simulink model "gm_HDL_pfc_gold_fi"  (R2024b)
settings: Solver=FixedStepDiscrete  StartTime=0.0  StopTime=.4  RelTol=1e-3
InitFcn:
  | fidelity_pfc_vals;
  | load('C:\Users\Angel\Desktop\hil\pfc3ph\matlab\sim\sschdl\pfc_desktop\stateSpaceParameters.mat');
undefined symbols (not defined in the file or in its folder): a, b, c, Down, tsw, Up
libraries: hdlmdlgenlib x24, simulink x23, hdlsllib x7, eePwmGenerator x3, dspsrcs4 x3, simulink_need_slupdate x1
(part 1 of 3)
settings Model: Creator=angro  LastModifiedBy=Angel
settings OptimizationCC: BlockReduction=off  ConditionallyExecuteInputs=off  DefaultParameterBehavior=Inlined  InheritOutputTypeSmallerThanSingle=on  DefaultUnderspecifiedDataType=single
settings DebuggingCC: SignalRangeChecking=warning  AlgebraicLoopMsg=error  ArtificialAlgebraicLoopMsg=error  InheritedTsInSrcMsg=none  SingleTaskRateTransMsg=error  UnconnectedInputMsg=warning  UnconnectedOutputMsg=warning  UnconnectedLineMsg=warning
settings HardwareCC: ProdBitPerPointer=32  ProdBitPerSizeT=32  ProdBitPerPtrDiffT=32  ProdLargestAtomicFloat=None  ProdIntDivRoundTo=Undefined  ProdEndianess=Unspecified  ProdWordSize=32  ProdHWDeviceType=ASIC/FPGA->ASIC/FPGA  TargetBitPerPointer=64  TargetBitPerSizeT=64  TargetBitPerPtrDiffT=64  TargetLongLongMode=on  TargetIntDivRoundTo=Zero  TargetEndianess=LittleEndian  TargetWordSize=64  TargetHWDeviceType=Custom Processor->MATLAB Host Computer  ProdEqTarget=off

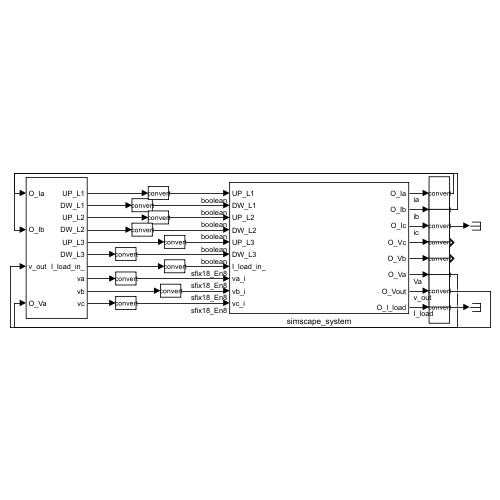
[thumbnail: Simulink's stored preview of the top-level diagram]
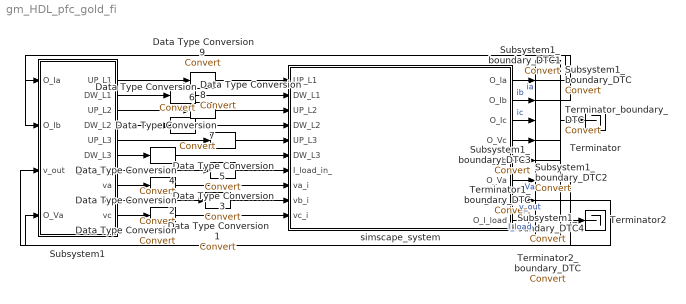
== system gm_HDL_pfc_gold_fi ==
  Data Type Conversion{,1..9} (10 alike) : DataTypeConversion  SaturateOnIntegerOverflow=off  RndMeth=Floor
  Subsystem1 : Subsystem
  Subsystem1_boundary_DTC{,1..4} (5 alike) : DataTypeConversion
  Terminator : Terminator
  Terminator1_boundary_DTC : DataTypeConversion
  Terminator2 : Terminator
  Terminator2_boundary_DTC : DataTypeConversion
  Terminator_boundary_DTC : DataTypeConversion
  simscape_system : Subsystem
  wires:
  Subsystem1_boundary_DTC4/1 -> Subsystem1/4(O_Va)
  Subsystem1_boundary_DTC1/1 -> Subsystem1/2(O_Ib)
  Subsystem1_boundary_DTC/1 -> Subsystem1/1(O_Ia)
  Terminator2_boundary_DTC/1 -> Terminator2/1
  simscape_system/8(O_I_load) -> Terminator2_boundary_DTC/1  "I_load"
  Terminator1_boundary_DTC/1 -> Subsystem1/3(v_out)
  simscape_system/7(O_Vout) -> Terminator1_boundary_DTC/1  "v_out"
  simscape_system/6(O_Va) -> Subsystem1_boundary_DTC4/1  "Va"
  simscape_system/5(O_Vb) -> Subsystem1_boundary_DTC3/1
  simscape_system/4(O_Vc) -> Subsystem1_boundary_DTC2/1
  Terminator_boundary_DTC/1 -> Terminator/1
  simscape_system/3(O_Ic) -> Terminator_boundary_DTC/1  "ic"
  simscape_system/2(O_Ib) -> Subsystem1_boundary_DTC1/1  "ib"
  simscape_system/1(O_Ia) -> Subsystem1_boundary_DTC/1  "ia"
  Data Type Conversion9/1 -> simscape_system/1(UP_L1)
  Data Type Conversion8/1 -> simscape_system/2(DW_L1)
  Data Type Conversion7/1 -> simscape_system/3(UP_L2)
  Data Type Conversion6/1 -> simscape_system/4(DW_L2)
  Data Type Conversion5/1 -> simscape_system/5(UP_L3)
  Data Type Conversion4/1 -> simscape_system/6(DW_L3)
  Data Type Conversion3/1 -> simscape_system/7(I_load_in_)
  Data Type Conversion2/1 -> simscape_system/8(va_i)
  Data Type Conversion1/1 -> simscape_system/9(vb_i)
  Data Type Conversion/1 -> simscape_system/10(vc_i)
  Subsystem1/10(vc) -> Data Type Conversion/1
  Subsystem1/9(vb) -> Data Type Conversion1/1
  Subsystem1/8(va) -> Data Type Conversion2/1
  Subsystem1/6(DW_L3) -> Data Type Conversion4/1
  Subsystem1/5(UP_L3) -> Data Type Conversion5/1
  Subsystem1/4(DW_L2) -> Data Type Conversion6/1
  Subsystem1/3(UP_L2) -> Data Type Conversion7/1
  Subsystem1/2(DW_L1) -> Data Type Conversion8/1
  Subsystem1/1(UP_L1) -> Data Type Conversion9/1
  Subsystem1/7(I_load_in_) -> Data Type Conversion3/1

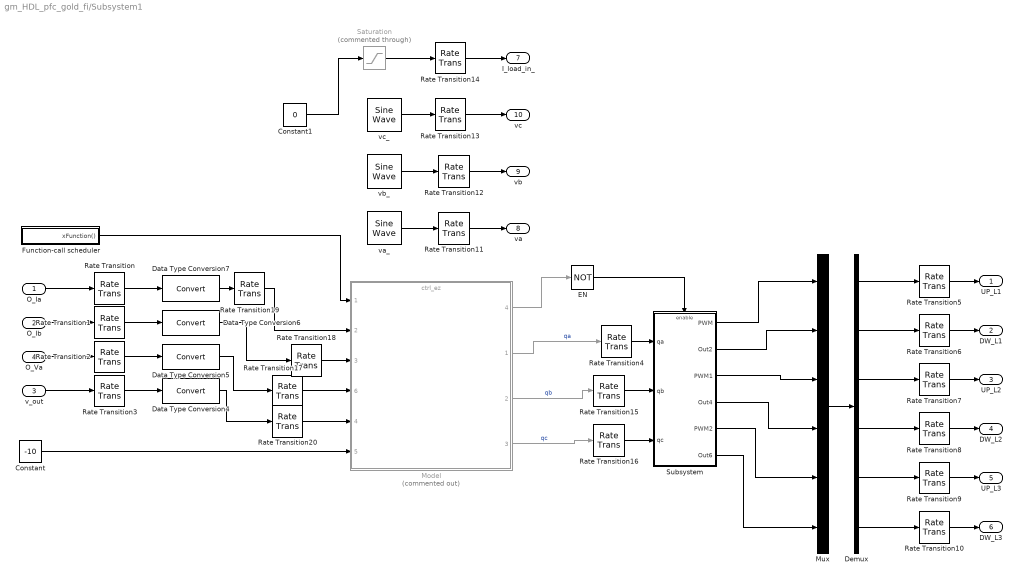
== system gm_HDL_pfc_gold_fi/Subsystem1 ==
  O_Ia : Inport
  O_Ib : Inport  Port=2
  v_out : Inport  Port=3
  O_Va : Inport  Port=4
  Constant : Constant  Value=-10  OutDataTypeStr=single  SampleTime=-1
  Constant1 : Constant  Value=0
  Data Type Conversion{4..7} (4 alike) : DataTypeConversion  SaturateOnIntegerOverflow=off  RndMeth=Floor
  Demux : Demux  Outputs=6
  EN : Logic  Operator=NOT  IconShape=distinctive  AllPortsSameDT=off  OutDataTypeStr=boolean
  Function-call scheduler : Test Sequence  TreatAsAtomicUnit=on  SystemSampleTime=tsw
  Model : ModelReference  Commented=on  ModelNameDialog=ctrl_ez.slx  SimulationMode=Normal  ScheduleRates=on  ModelReferenceVersion=1.93
      settings: PortSchema="{\"entries\":[{\"content\":{\"sides\":[{\"content\":{\"connectorIds\":[\"In1\",\"In2\",\"In3\",\"In6\",\"In4\",\"In5\"]},\"type\":\"ConnectorPlacement.EquallySpacedRectSide\",\"uuid\":\"06228333-cac0-4194-8a9e-b8aeb0f2d2c3\"},{\"content\":{\"connectorIds\":[\"Out4\",\"Out1\",\"Out2\",\"Out3\"],\"side\":\"RIGHT\"},\"type\":\"ConnectorPlacement.EquallySpacedRectSide\",\"uuid\":\"40fc62da-d5d1-4d07-aeb6-22788cb15ec8\"},{\"content\":{\"side\":\"TOP\"},\"type\":\"ConnectorPlacement.EquallySpacedRectSide\",\"uuid\":\"88200490-c98c-4a0a-a21b-c8f9cef9ee2d\"}]},\"type\":\"ConnectorPlacement.EquallySpacedConnector\",\"uuid\":\"5f40978a-c38c-41d1-a6a1-03264eebf395\"}],\"packageUris\":[\"http://schema.mathworks.com/mf0/Connector/R2020b\"],\"version\":\"1.0\"}"
  Mux : Mux  Inputs=6
  Rate Transition{,1..3,14} (5 alike) : RateTransition  OutPortSampleTime=t_ss
  Rate Transition{4..13,15..20} (16 alike) : RateTransition
  Saturation : Saturate  Commented=through  UpperLimit=3
  Subsystem : Subsystem
  va_ : dspsrcs4/Sine Wave  Amplitude=325  Frequency=50  Phase=0  SampleMode=Discrete  OutComplex=Real  CompMethod=Table lookup  TableSize=Speed  SampleTime=tsw  SamplesPerFrame=1  ResetState=Restart at time zero  OutputFrames=off  dataType=double  wordLen=16  udDataType=sfix(16)  fracBitsMode=Best precision  numFracBits=15  OutDataTypeStr=double  LastOutDataTypeStr=double
  vb_ : dspsrcs4/Sine Wave  Amplitude=325  Frequency=50  Phase=(-2*pi/3)  SampleMode=Discrete  OutComplex=Real  CompMethod=Table lookup  TableSize=Speed  SampleTime=tsw  SamplesPerFrame=1  ResetState=Restart at time zero  OutputFrames=off  dataType=double  wordLen=16  udDataType=sfix(16)  fracBitsMode=Best precision  numFracBits=15  OutDataTypeStr=double  LastOutDataTypeStr=double
  vc_ : dspsrcs4/Sine Wave  Amplitude=325  Frequency=50  Phase=(2*pi/3)  SampleMode=Discrete  OutComplex=Real  CompMethod=Table lookup  TableSize=Speed  SampleTime=tsw  SamplesPerFrame=1  ResetState=Restart at time zero  OutputFrames=off  dataType=double  wordLen=16  udDataType=sfix(16)  fracBitsMode=Best precision  numFracBits=15  OutDataTypeStr=double  LastOutDataTypeStr=double
  UP_L1 : Outport
  DW_L1 : Outport  Port=2
  UP_L2 : Outport  Port=3
  DW_L2 : Outport  Port=4
  UP_L3 : Outport  Port=5
  DW_L3 : Outport  Port=6
  I_load_in_ : Outport  Port=7
  va : Outport  Port=8
  vb : Outport  Port=9
  vc : Outport  Port=10
  wires:
  Rate Transition20/1 -> Model/4
  Rate Transition17/1 -> Model/6
  Rate Transition18/1 -> Model/3
  Rate Transition19/1 -> Model/2
  Rate Transition16/1 -> Subsystem/3(qc)
  Rate Transition15/1 -> Subsystem/2(qb)
  Rate Transition4/1 -> Subsystem/1(qa)
  EN/1 -> Subsystem/Enable
  Model/4 -> EN/1
  Subsystem/6(Out6) -> Mux/6
  Subsystem/5(PWM2) -> Mux/5
  Subsystem/4(Out4) -> Mux/4
  Subsystem/3(PWM1) -> Mux/3
  Subsystem/2(Out2) -> Mux/2
  Subsystem/1(PWM) -> Mux/1
  Model/3 -> Rate Transition16/1  "qc"
  Model/2 -> Rate Transition15/1  "qb"
  Model/1 -> Rate Transition4/1  "qa"
  Mux/1 -> Demux/1
  Function-call scheduler/1(xFunction()) -> Model/1
  Constant1/1 -> Saturation/1
  Constant/1 -> Model/5
  Data Type Conversion4/1 -> Rate Transition20/1
  Data Type Conversion5/1 -> Rate Transition17/1
  Data Type Conversion6/1 -> Rate Transition18/1
  Data Type Conversion7/1 -> Rate Transition19/1
  Rate Transition2/1 -> Data Type Conversion5/1
  Rate Transition1/1 -> Data Type Conversion6/1
  Rate Transition/1 -> Data Type Conversion7/1
  Rate Transition3/1 -> Data Type Conversion4/1
  Rate Transition7/1 -> UP_L2/1
  Demux/6 -> Rate Transition10/1
  Demux/2 -> Rate Transition6/1
  Demux/1 -> Rate Transition5/1
  Rate Transition5/1 -> UP_L1/1
  Rate Transition9/1 -> UP_L3/1
  Rate Transition13/1 -> vc/1
  Rate Transition8/1 -> DW_L2/1
  Demux/3 -> Rate Transition7/1
  Demux/4 -> Rate Transition8/1
  Rate Transition11/1 -> va/1
  Demux/5 -> Rate Transition9/1
  va_/1 -> Rate Transition11/1
  vc_/1 -> Rate Transition13/1
  v_out/1 -> Rate Transition3/1
  Rate Transition6/1 -> DW_L1/1
  vb_/1 -> Rate Transition12/1
  O_Ib/1 -> Rate Transition1/1
  Rate Transition12/1 -> vb/1
  O_Va/1 -> Rate Transition2/1
  O_Ia/1 -> Rate Transition/1
  Rate Transition14/1 -> I_load_in_/1
  Rate Transition10/1 -> DW_L3/1
  Saturation/1 -> Rate Transition14/1

== system gm_HDL_pfc_gold_fi/simscape_system ==
  UP_L1 : Inport  OutDataTypeStr=boolean  PortDimensions=1  SampleTime=5.12820512820513e-07
  DW_L1 : Inport  Port=2  OutDataTypeStr=boolean  PortDimensions=1  SampleTime=5.12820512820513e-07
  UP_L2 : Inport  Port=3  OutDataTypeStr=boolean  PortDimensions=1  SampleTime=5.12820512820513e-07
  DW_L2 : Inport  Port=4  OutDataTypeStr=boolean  PortDimensions=1  SampleTime=5.12820512820513e-07
  UP_L3 : Inport  Port=5  OutDataTypeStr=boolean  PortDimensions=1  SampleTime=5.12820512820513e-07
  DW_L3 : Inport  Port=6  OutDataTypeStr=boolean  PortDimensions=1  SampleTime=5.12820512820513e-07
  I_load_in_ : Inport  Port=7  OutDataTypeStr=fixdt(1, 18, 8)  PortDimensions=1  SampleTime=5.12820512820513e-07
  va_i : Inport  Port=8  OutDataTypeStr=fixdt(1, 18, 8)  PortDimensions=1  SampleTime=5.12820512820513e-07  LockScale=on
  vb_i : Inport  Port=9  OutDataTypeStr=fixdt(1, 18, 8)  PortDimensions=1  SampleTime=5.12820512820513e-07  LockScale=on
  vc_i : Inport  Port=10  OutDataTypeStr=fixdt(1, 18, 8)  PortDimensions=1  SampleTime=5.12820512820513e-07  LockScale=on
  simscape_system : Subsystem
  t{,1..7} (8 alike) : RateTransition  InitialCondition=double(0)  OutPortSampleTimeOpt=Multiple of input port sample time  OutPortSampleTimeMultiple=67
  O_Ia : Outport  SampleTime=5.12820512820513e-07
  O_Ib : Outport  Port=2  SampleTime=5.12820512820513e-07
  O_Ic : Outport  Port=3  SampleTime=5.12820512820513e-07
  O_Vc : Outport  Port=4  SampleTime=5.12820512820513e-07
  O_Vb : Outport  Port=5  SampleTime=5.12820512820513e-07
  O_Va : Outport  Port=6  SampleTime=5.12820512820513e-07
  O_Vout : Outport  Port=7  SampleTime=5.12820512820513e-07
  O_I_load : Outport  Port=8  SampleTime=5.12820512820513e-07
  wires:
  UP_L1/1 -> simscape_system/1(UP_L1)
  t1/1 -> O_Ic/1
  DW_L1/1 -> simscape_system/2(DW_L1)
  UP_L2/1 -> simscape_system/3(UP_L2)
  va_i/1 -> simscape_system/8(va_i)
  I_load_in_/1 -> simscape_system/7(I_load_in_)
  simscape_system/1(O_Ia) -> t7/1
  DW_L2/1 -> simscape_system/4(DW_L2)
  UP_L3/1 -> simscape_system/5(UP_L3)
  DW_L3/1 -> simscape_system/6(DW_L3)
  vb_i/1 -> simscape_system/9(vb_i)
  vc_i/1 -> simscape_system/10(vc_i)
  simscape_system/2(O_Ib) -> t/1
  t6/1 -> O_I_load/1
  simscape_system/3(O_Ic) -> t1/1
  simscape_system/4(O_Vc) -> t2/1
  simscape_system/5(O_Vb) -> t3/1
  simscape_system/6(O_Va) -> t4/1
  simscape_system/7(O_Vout) -> t5/1
  simscape_system/8(O_I_load) -> t6/1
  t7/1 -> O_Ia/1
  t/1 -> O_Ib/1
  t2/1 -> O_Vc/1
  t3/1 -> O_Vb/1
  t4/1 -> O_Va/1
  t5/1 -> O_Vout/1

== system gm_HDL_pfc_gold_fi/Subsystem1/Subsystem ==
  qa : Inport
  qb : Inport  Port=2
  qc : Inport  Port=3
  Enable : EnablePort
  NOT : Logic  Operator=NOT  IconShape=distinctive  AllPortsSameDT=off  OutDataTypeStr=boolean
  NOT1 : Logic  Operator=NOT  IconShape=distinctive  AllPortsSameDT=off  OutDataTypeStr=boolean
  NOT2 : Logic  Operator=NOT  IconShape=distinctive  AllPortsSameDT=off  OutDataTypeStr=boolean
  PWM Generator : eePwmGenerator/PWM Generator  CarrCount=Up-Down  Tper=tsw  Tdelay=0  Ts=tsw/10
  PWM Generator1 : eePwmGenerator/PWM Generator  CarrCount=Up-Down  Tper=tsw  Tdelay=0  Ts=tsw/10
  PWM Generator2 : eePwmGenerator/PWM Generator  CarrCount=Up-Down  Tper=tsw  Tdelay=0  Ts=tsw/10
  PWM : Outport
  Out2 : Outport  Port=2
  PWM1 : Outport  Port=3
  Out4 : Outport  Port=4
  PWM2 : Outport  Port=5
  Out6 : Outport  Port=6
  wires:
  qb/1 -> PWM Generator1/1
  NOT2/1 -> Out6/1
  NOT/1 -> Out2/1
  NOT1/1 -> Out4/1
  PWM Generator1/1 -> NOT1/1, PWM1/1
  qa/1 -> PWM Generator/1
  PWM Generator/1 -> NOT/1, PWM/1
  qc/1 -> PWM Generator2/1
  PWM Generator2/1 -> PWM2/1, NOT2/1

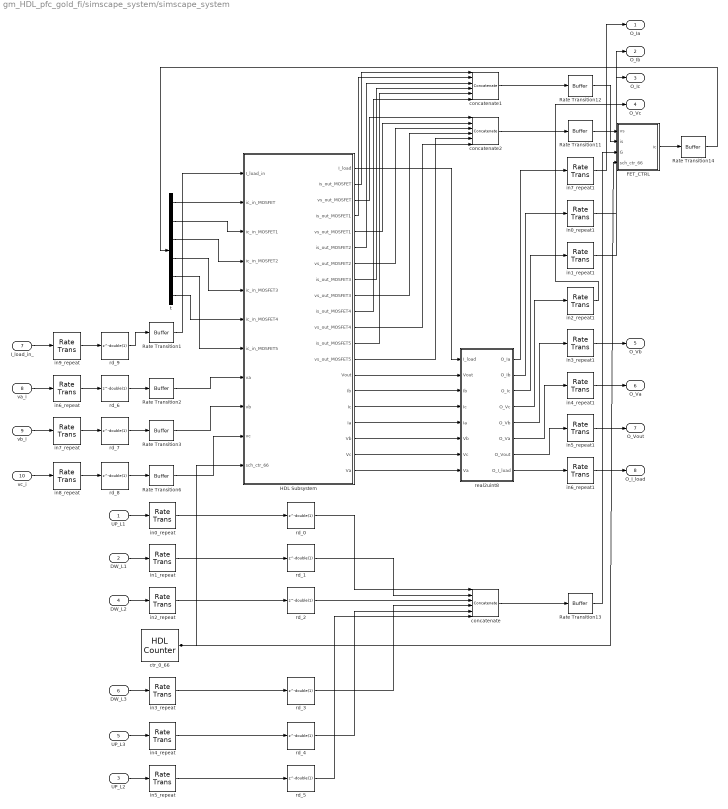
== system gm_HDL_pfc_gold_fi/simscape_system/simscape_system ==
  UP_L1 : Inport  OutDataTypeStr=boolean  SampleTime=5.12820512820513e-07
  DW_L1 : Inport  Port=2  OutDataTypeStr=boolean  SampleTime=5.12820512820513e-07
  UP_L2 : Inport  Port=3  OutDataTypeStr=boolean  SampleTime=5.12820512820513e-07
  DW_L2 : Inport  Port=4  OutDataTypeStr=boolean  SampleTime=5.12820512820513e-07
  UP_L3 : Inport  Port=5  OutDataTypeStr=boolean  SampleTime=5.12820512820513e-07
  DW_L3 : Inport  Port=6  OutDataTypeStr=boolean  SampleTime=5.12820512820513e-07
  I_load_in_ : Inport  Port=7  OutDataTypeStr=fixdt(1, 18, 8)  SampleTime=5.12820512820513e-07
  va_i : Inport  Port=8  OutDataTypeStr=fixdt(1, 18, 8)  SampleTime=5.12820512820513e-07
  vb_i : Inport  Port=9  OutDataTypeStr=fixdt(1, 18, 8)  SampleTime=5.12820512820513e-07
  vc_i : Inport  Port=10  OutDataTypeStr=fixdt(1, 18, 8)  SampleTime=5.12820512820513e-07
  FET_CTRL : Subsystem
  HDL Subsystem : Subsystem
  Rate Transition{1..3,6,11..14} (8 alike) : hdlmdlgenlib/Buffer
  concatenate : Concatenate  NumInputs=6
  concatenate1 : Concatenate  NumInputs=6
  concatenate2 : Concatenate  NumInputs=6
  ctr_0_66 : hdlsllib/Sources/HDL Counter  CountType=Count limited  CountInit=double(0)  CountStep=double(1)  CountMax=double(66)  CountFromType=Initial value  CountFrom=double(0)  CountResetPort=off  CountLoadPort=off  CountEnbPort=off  CountDirPort=off  CountHitOutputPort=off  CountDataType=Unsigned  CountWordLen=7  CountFracLen=0  CountSampTime=7.65403750478377e-09
  in0_repeat : RateTransition  Integrity=off  Deterministic=off  OutPortSampleTimeOpt=Multiple of input port sample time  OutPortSampleTimeMultiple=1/67
  in0_repeat1 : RateTransition  Integrity=off  Deterministic=off  OutPortSampleTimeOpt=Multiple of input port sample time  OutPortSampleTimeMultiple=1/67
  in1_repeat : RateTransition  Integrity=off  Deterministic=off  OutPortSampleTimeOpt=Multiple of input port sample time  OutPortSampleTimeMultiple=1/67
  in1_repeat1 : RateTransition  Integrity=off  Deterministic=off  OutPortSampleTimeOpt=Multiple of input port sample time  OutPortSampleTimeMultiple=1/67
  in2_repeat : RateTransition  Integrity=off  Deterministic=off  OutPortSampleTimeOpt=Multiple of input port sample time  OutPortSampleTimeMultiple=1/67
  in2_repeat1 : RateTransition  Integrity=off  Deterministic=off  OutPortSampleTimeOpt=Multiple of input port sample time  OutPortSampleTimeMultiple=1/67
  in3_repeat : RateTransition  Integrity=off  Deterministic=off  OutPortSampleTimeOpt=Multiple of input port sample time  OutPortSampleTimeMultiple=1/67
  in3_repeat1 : RateTransition  Integrity=off  Deterministic=off  OutPortSampleTimeOpt=Multiple of input port sample time  OutPortSampleTimeMultiple=1/67
  in4_repeat : RateTransition  Integrity=off  Deterministic=off  OutPortSampleTimeOpt=Multiple of input port sample time  OutPortSampleTimeMultiple=1/67
  in4_repeat1 : RateTransition  Integrity=off  Deterministic=off  OutPortSampleTimeOpt=Multiple of input port sample time  OutPortSampleTimeMultiple=1/67
  in5_repeat : RateTransition  Integrity=off  Deterministic=off  OutPortSampleTimeOpt=Multiple of input port sample time  OutPortSampleTimeMultiple=1/67
  in5_repeat1 : RateTransition  Integrity=off  Deterministic=off  OutPortSampleTimeOpt=Multiple of input port sample time  OutPortSampleTimeMultiple=1/67
  in6_repeat : RateTransition  Integrity=off  Deterministic=off  OutPortSampleTimeOpt=Multiple of input port sample time  OutPortSampleTimeMultiple=1/67
  in6_repeat1 : RateTransition  Integrity=off  Deterministic=off  OutPortSampleTimeOpt=Multiple of input port sample time  OutPortSampleTimeMultiple=1/67
  in7_repeat : RateTransition  Integrity=off  Deterministic=off  OutPortSampleTimeOpt=Multiple of input port sample time  OutPortSampleTimeMultiple=1/67
  in7_repeat1 : RateTransition  Integrity=off  Deterministic=off  OutPortSampleTimeOpt=Multiple of input port sample time  OutPortSampleTimeMultiple=1/67
  in8_repeat : RateTransition  Integrity=off  Deterministic=off  OutPortSampleTimeOpt=Multiple of input port sample time  OutPortSampleTimeMultiple=1/67
  in9_repeat : RateTransition  Integrity=off  Deterministic=off  OutPortSampleTimeOpt=Multiple of input port sample time  OutPortSampleTimeMultiple=1/67
  rd_{0..9} (10 alike) : Delay  DelayLength=double(1)  InitialCondition=0  SampleTime=7.65403750478377e-09
  real2uint8 : Subsystem
  t : Demux  Outputs=6
  O_Ia : Outport  OutDataTypeStr=uint8  SampleTime=7.65403750478377e-09
  O_Ib : Outport  Port=2  OutDataTypeStr=uint8  SampleTime=7.65403750478377e-09
  O_Ic : Outport  Port=3  OutDataTypeStr=uint8  SampleTime=7.65403750478377e-09
  O_Vc : Outport  Port=4  OutDataTypeStr=uint8  SampleTime=7.65403750478377e-09
  O_Vb : Outport  Port=5  OutDataTypeStr=uint8  SampleTime=7.65403750478377e-09
  O_Va : Outport  Port=6  OutDataTypeStr=uint8  SampleTime=7.65403750478377e-09
  O_Vout : Outport  Port=7  OutDataTypeStr=uint8  SampleTime=7.65403750478377e-09
  O_I_load : Outport  Port=8  OutDataTypeStr=uint8  SampleTime=7.65403750478377e-09
  wires:
  t/1 -> HDL Subsystem/2(ic_in_MOSFET)
  real2uint8/8(O_I_load) -> in6_repeat1/1
  I_load_in_/1 -> in9_repeat/1
  in8_repeat/1 -> rd_8/1
  vc_i/1 -> in8_repeat/1
  va_i/1 -> in6_repeat/1
  HDL Subsystem/6(is_out_MOSFET2) -> concatenate1/3
  in7_repeat/1 -> rd_7/1
  HDL Subsystem/12(is_out_MOSFET5) -> concatenate1/5
  HDL Subsystem/4(is_out_MOSFET1) -> concatenate1/2
  DW_L1/1 -> in1_repeat/1
  vb_i/1 -> in7_repeat/1
  in4_repeat1/1 -> O_Va/1
  in9_repeat/1 -> rd_9/1
  HDL Subsystem/19(Vc) -> real2uint8/7(Vc)
  rd_7/1 -> Rate Transition3/1
  in6_repeat/1 -> rd_6/1
  rd_9/1 -> Rate Transition1/1
  rd_6/1 -> Rate Transition2/1
  in2_repeat/1 -> rd_2/1
  rd_8/1 -> Rate Transition6/1
  UP_L3/1 -> in4_repeat/1
  UP_L1/1 -> in0_repeat/1
  HDL Subsystem/18(Vb) -> real2uint8/6(Vb)
  in1_repeat/1 -> rd_1/1
  t/3 -> HDL Subsystem/4(ic_in_MOSFET2)
  DW_L2/1 -> in2_repeat/1
  HDL Subsystem/14(Vout) -> real2uint8/2(Vout)
  DW_L3/1 -> in3_repeat/1
  UP_L2/1 -> in5_repeat/1
  t/2 -> HDL Subsystem/3(ic_in_MOSFET1)
  t/4 -> HDL Subsystem/5(ic_in_MOSFET3)
  concatenate2/1 -> Rate Transition11/1
  HDL Subsystem/8(is_out_MOSFET3) -> concatenate1/4
  concatenate1/1 -> Rate Transition12/1
  real2uint8/1(O_Ia) -> in7_repeat1/1
  t/5 -> HDL Subsystem/7(ic_in_MOSFET5)
  HDL Subsystem/16(Ic) -> real2uint8/4(Ic)
  t/6 -> HDL Subsystem/6(ic_in_MOSFET4)
  Rate Transition1/1 -> HDL Subsystem/1(I_load_in)
  Rate Transition2/1 -> HDL Subsystem/8(va)
  in5_repeat/1 -> rd_5/1
  Rate Transition3/1 -> HDL Subsystem/9(vb)
  in3_repeat/1 -> rd_3/1
  Rate Transition6/1 -> HDL Subsystem/10(vc)
  real2uint8/6(O_Va) -> in4_repeat1/1
  in0_repeat/1 -> rd_0/1
  ctr_0_66/1 -> FET_CTRL/4(sch_ctr_66), HDL Subsystem/11(sch_ctr_66)
  in4_repeat/1 -> rd_4/1
  rd_0/1 -> concatenate/1
  HDL Subsystem/1(I_load) -> real2uint8/1(I_load)
  HDL Subsystem/17(Ia) -> real2uint8/5(Ia)
  HDL Subsystem/2(is_out_MOSFET) -> concatenate1/1
  HDL Subsystem/11(vs_out_MOSFET4) -> concatenate2/6
  HDL Subsystem/3(vs_out_MOSFET) -> concatenate2/1
  HDL Subsystem/5(vs_out_MOSFET1) -> concatenate2/2
  HDL Subsystem/7(vs_out_MOSFET2) -> concatenate2/3
  HDL Subsystem/9(vs_out_MOSFET3) -> concatenate2/4
  HDL Subsystem/10(is_out_MOSFET4) -> concatenate1/6
  HDL Subsystem/13(vs_out_MOSFET5) -> concatenate2/5
  HDL Subsystem/20(Va) -> real2uint8/8(Va)
  HDL Subsystem/15(Ib) -> real2uint8/3(Ib)
  rd_1/1 -> concatenate/2
  rd_2/1 -> concatenate/3
  rd_3/1 -> concatenate/4
  rd_4/1 -> concatenate/5
  rd_5/1 -> concatenate/6
  real2uint8/2(O_Ib) -> in0_repeat1/1
  real2uint8/3(O_Ic) -> in1_repeat1/1
  real2uint8/4(O_Vc) -> in2_repeat1/1
  real2uint8/5(O_Vb) -> in3_repeat1/1
  real2uint8/7(O_Vout) -> in5_repeat1/1
  concatenate/1 -> Rate Transition13/1
  Rate Transition12/1 -> FET_CTRL/2(is)
  Rate Transition11/1 -> FET_CTRL/1(vs)
  in7_repeat1/1 -> O_Ia/1
  in0_repeat1/1 -> O_Ib/1
  in1_repeat1/1 -> O_Ic/1
  in2_repeat1/1 -> O_Vc/1
  in3_repeat1/1 -> O_Vb/1
  in5_repeat1/1 -> O_Vout/1
  in6_repeat1/1 -> O_I_load/1
  Rate Transition13/1 -> FET_CTRL/3(G)
  FET_CTRL/1(ic) -> Rate Transition14/1
  Rate Transition14/1 -> t/1

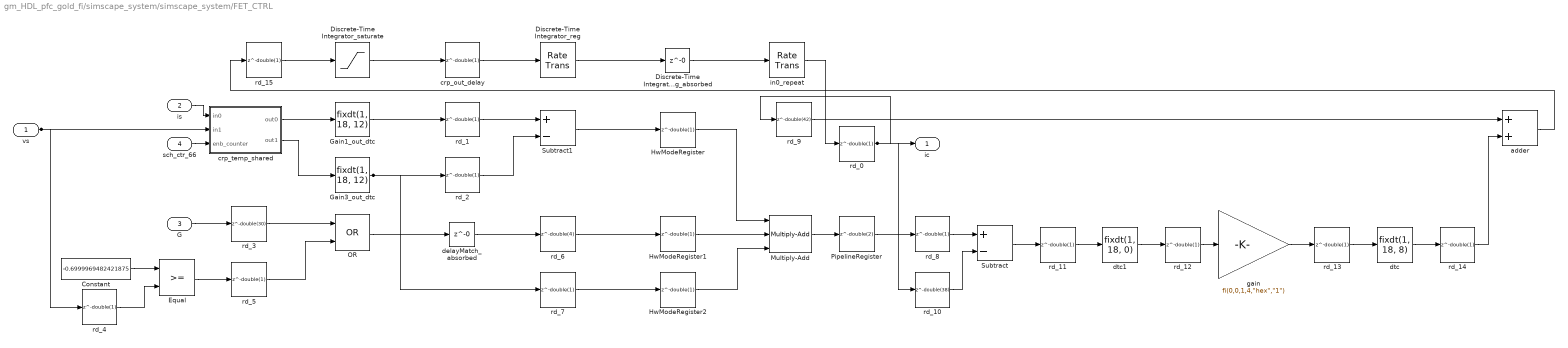
== system gm_HDL_pfc_gold_fi/simscape_system/simscape_system/FET_CTRL ==
  vs : Inport  OutDataTypeStr=fixdt(1, 18, 6)  PortDimensions=[6]  SampleTime=7.65403750478377e-09
  is : Inport  Port=2  OutDataTypeStr=fixdt(1, 18, 6)  PortDimensions=[6]  SampleTime=7.65403750478377e-09
  G : Inport  Port=3  OutDataTypeStr=boolean  PortDimensions=[6]  SampleTime=7.65403750478377e-09
  sch_ctr_66 : Inport  Port=4  OutDataTypeStr=fixdt(0, 7, 0)  SampleTime=7.65403750478377e-09
  Constant : Constant  Value=-0.6999969482421875  OutDataTypeStr=fixdt(1, 18, 17)  SampleTime=7.65403750478377e-09
  Discrete-Time Integrator_reg : RateTransition  InitialCondition=double(0)  OutPortSampleTimeOpt=Multiple of input port sample time  OutPortSampleTimeMultiple=67
  Discrete-Time Integrator_reg_absorbed : Delay  DelayLength=0
  Discrete-Time Integrator_saturate : Saturate  UpperLimit="fi(0,1,18,8,\"hex\",\"06400\")"  LowerLimit="fi(0,1,18,8,\"hex\",\"39c00\")"  SampleTime=7.65403750478377e-09  OutDataTypeStr=fixdt(1, 18, 8)
  Equal : RelationalOperator  OutDataTypeStr=boolean  SampleTime=7.65403750478377e-09  InputSameDT=off
  Gain1_out_dtc : DataTypeConversion  OutDataTypeStr=fixdt(1, 18, 12)  SampleTime=7.65403750478377e-09  SaturateOnIntegerOverflow=off  RndMeth=Floor
  Gain3_out_dtc : DataTypeConversion  OutDataTypeStr=fixdt(1, 18, 12)  SampleTime=7.65403750478377e-09  SaturateOnIntegerOverflow=off  RndMeth=Floor
  HwModeRegister : Delay  DelayLength=double(1)  InitialCondition=0  SampleTime=7.65403750478377e-09
  HwModeRegister1 : Delay  DelayLength=double(1)  InitialCondition=0  SampleTime=7.65403750478377e-09
  HwModeRegister2 : Delay  DelayLength=double(1)  InitialCondition=0  SampleTime=7.65403750478377e-09
  Multiply-Add : hdlsllib/HDL Operations/Multiply-Add  Function=c+(a.*b)  datatype=fixdt(1, 18, 12)  DoSatur=on  FMA=off
  OR : Logic  Operator=OR  AllPortsSameDT=off  OutDataTypeStr=boolean  SampleTime=7.65403750478377e-09
  PipelineRegister : Delay  DelayLength=double(2)  InitialCondition=0  SampleTime=7.65403750478377e-09
  Subtract : Sum  Inputs=+-  OutDataTypeStr=fixdt(1, 18, 12)  AccumDataTypeStr=fixdt(1, 23, 12)  SampleTime=7.65403750478377e-09
  Subtract1 : Sum  Inputs=+-  OutDataTypeStr=fixdt(1, 18, 11)  AccumDataTypeStr=fixdt(1, 19, 12)  SampleTime=7.65403750478377e-09
  adder : Sum  OutDataTypeStr=fixdt(1, 18, 8)  AccumDataTypeStr=fixdt(1, 18, 8)  SaturateOnIntegerOverflow=on  SampleTime=7.65403750478377e-09
  crp_out_delay : Delay  DelayLength=double(1)  InitialCondition=0  SampleTime=7.65403750478377e-09
  crp_temp_shared : Subsystem
  delayMatch_absorbed : Delay  DelayLength=0
  dtc : DataTypeConversion  OutDataTypeStr=fixdt(1, 18, 8)  ConvertRealWorld=Stored Integer (SI)  SampleTime=7.65403750478377e-09  RndMeth=Floor
  dtc1 : DataTypeConversion  OutDataTypeStr=fixdt(1, 18, 0)  ConvertRealWorld=Stored Integer (SI)  SampleTime=7.65403750478377e-09  RndMeth=Floor
  gain : Gain  Gain="fi(0,0,1,4,\"hex\",\"1\")"  ParamDataTypeStr=fixdt(0, 1, 4)  OutDataTypeStr=fixdt(1, 18, 0)  SaturateOnIntegerOverflow=on  SampleTime=7.65403750478377e-09
  in0_repeat : RateTransition  Integrity=off  Deterministic=off  OutPortSampleTimeOpt=Multiple of input port sample time  OutPortSampleTimeMultiple=1/67
  rd_{0..2,4..5,7..8,11..15} (12 alike) : Delay  DelayLength=double(1)  InitialCondition=0  SampleTime=7.65403750478377e-09
  rd_10 : Delay  DelayLength=double(38)  InitialCondition=0  SampleTime=7.65403750478377e-09
  rd_3 : Delay  DelayLength=double(30)  InitialCondition=0  SampleTime=7.65403750478377e-09
  rd_6 : Delay  DelayLength=double(4)  InitialCondition=0  SampleTime=7.65403750478377e-09
  rd_9 : Delay  DelayLength=double(42)  InitialCondition=0  SampleTime=7.65403750478377e-09
  ic : Outport  SampleTime=7.65403750478377e-09
  wires:
  rd_10/1 -> Subtract/2
  vs/1 -> crp_temp_shared/2(in1), rd_4/1
  rd_15/1 -> Discrete-Time Integrator_saturate/1
  HwModeRegister2/1 -> Multiply-Add/3
  Constant/1 -> Equal/1
  rd_4/1 -> Equal/2
  rd_12/1 -> gain/1
  G/1 -> rd_3/1
  sch_ctr_66/1 -> crp_temp_shared/3(enb_counter)
  is/1 -> crp_temp_shared/1(in0)
  Equal/1 -> rd_5/1
  crp_temp_shared/1(out0) -> Gain1_out_dtc/1
  Subtract/1 -> rd_11/1
  OR/1 -> delayMatch_absorbed/1
  crp_temp_shared/2(out1) -> Gain3_out_dtc/1
  rd_3/1 -> OR/1
  dtc/1 -> rd_14/1
  rd_5/1 -> OR/2
  Discrete-Time Integrator_saturate/1 -> crp_out_delay/1
  rd_11/1 -> dtc1/1
  Gain1_out_dtc/1 -> rd_1/1
  Gain3_out_dtc/1 -> rd_7/1, rd_2/1
  crp_out_delay/1 -> Discrete-Time Integrator_reg/1
  Subtract1/1 -> HwModeRegister/1
  rd_1/1 -> Subtract1/1
  Discrete-Time Integrator_reg/1 -> Discrete-Time Integrator_reg_absorbed/1
  rd_2/1 -> Subtract1/2
  delayMatch_absorbed/1 -> rd_6/1
  Multiply-Add/1 -> PipelineRegister/1
  rd_6/1 -> HwModeRegister1/1
  rd_7/1 -> HwModeRegister2/1
  gain/1 -> rd_13/1
  Discrete-Time Integrator_reg_absorbed/1 -> in0_repeat/1
  HwModeRegister/1 -> Multiply-Add/1
  rd_0/1 -> rd_9/1, rd_10/1, ic/1
  HwModeRegister1/1 -> Multiply-Add/2
  in0_repeat/1 -> rd_0/1
  rd_9/1 -> adder/1
  PipelineRegister/1 -> rd_8/1
  rd_8/1 -> Subtract/1
  dtc1/1 -> rd_12/1
  rd_13/1 -> dtc/1
  rd_14/1 -> adder/2
  adder/1 -> rd_15/1

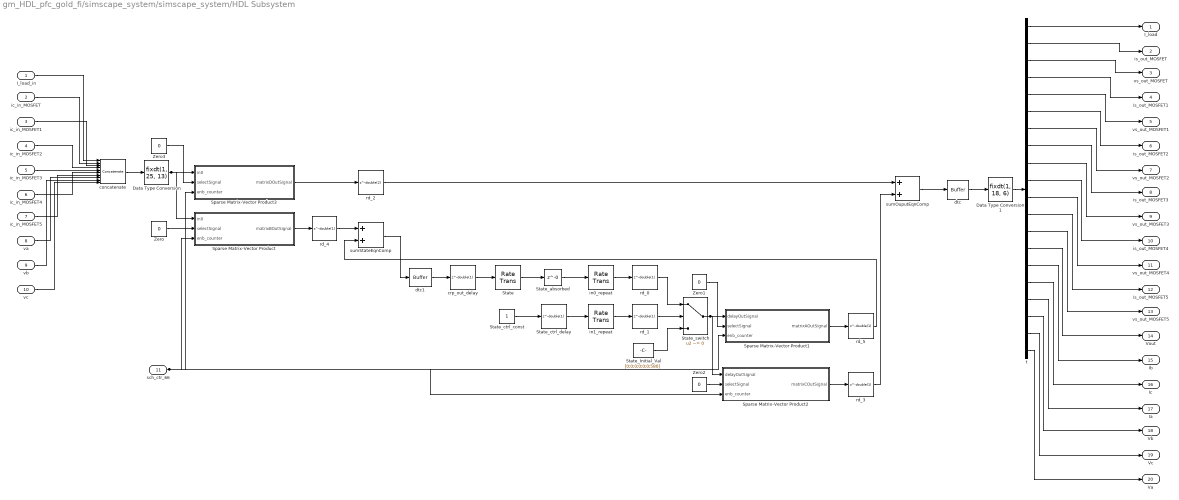
== system gm_HDL_pfc_gold_fi/simscape_system/simscape_system/HDL Subsystem ==
  I_load_in : Inport  OutDataTypeStr=fixdt(1, 18, 8)  PortDimensions=1  SampleTime=7.65403750478377e-09
  ic_in_MOSFET : Inport  Port=2  OutDataTypeStr=fixdt(1, 18, 8)  PortDimensions=1  SampleTime=7.65403750478377e-09
  ic_in_MOSFET1 : Inport  Port=3  OutDataTypeStr=fixdt(1, 18, 8)  PortDimensions=1  SampleTime=7.65403750478377e-09
  ic_in_MOSFET2 : Inport  Port=4  OutDataTypeStr=fixdt(1, 18, 8)  PortDimensions=1  SampleTime=7.65403750478377e-09
  ic_in_MOSFET3 : Inport  Port=5  OutDataTypeStr=fixdt(1, 18, 8)  PortDimensions=1  SampleTime=7.65403750478377e-09
  ic_in_MOSFET4 : Inport  Port=6  OutDataTypeStr=fixdt(1, 18, 8)  PortDimensions=1  SampleTime=7.65403750478377e-09
  ic_in_MOSFET5 : Inport  Port=7  OutDataTypeStr=fixdt(1, 18, 8)  PortDimensions=1  SampleTime=7.65403750478377e-09
  va : Inport  Port=8  OutDataTypeStr=fixdt(1, 18, 8)  PortDimensions=1  SampleTime=7.65403750478377e-09
  vb : Inport  Port=9  OutDataTypeStr=fixdt(1, 18, 8)  PortDimensions=1  SampleTime=7.65403750478377e-09
  vc : Inport  Port=10  OutDataTypeStr=fixdt(1, 18, 8)  PortDimensions=1  SampleTime=7.65403750478377e-09
  sch_ctr_66 : Inport  Port=11  OutDataTypeStr=fixdt(0, 7, 0)  SampleTime=7.65403750478377e-09
  Data Type Conversion : DataTypeConversion  OutDataTypeStr=fixdt(1, 25, 13)  SampleTime=7.65403750478377e-09  SaturateOnIntegerOverflow=off  RndMeth=Floor
  Data Type Conversion1 : DataTypeConversion  OutDataTypeStr=fixdt(1, 18, 6)  SampleTime=7.65403750478377e-09  SaturateOnIntegerOverflow=off  RndMeth=Floor
  Sparse Matrix-Vector Product : Subsystem
  Sparse Matrix-Vector Product1 : Subsystem
  Sparse Matrix-Vector Product2 : Subsystem
  Sparse Matrix-Vector Product3 : Subsystem
  State : RateTransition  InitialCondition=double(0)  OutPortSampleTimeOpt=Multiple of input port sample time  OutPortSampleTimeMultiple=67
  State_Initial_Val : Constant  Value=[0;0;0;0;0;0;580]  OutDataTypeStr=fixdt(1, 25, 13)  SampleTime=7.65403750478377e-09
  State_absorbed : Delay  DelayLength=0
  State_ctrl_const : Constant  OutDataTypeStr=boolean  SampleTime=5.12820512820513e-07
  State_ctrl_delay : Delay  DelayLength=double(1)  InitialCondition=0  SampleTime=5.12820512820513e-07
  State_switch : Switch  Criteria=u2 ~= 0  Threshold=double(0)  OutDataTypeStr=fixdt(1, 25, 13)  SampleTime=7.65403750478377e-09  SaturateOnIntegerOverflow=off  InputSameDT=off
  Zero{,1..3} (4 alike) : Constant  Value=0  OutDataTypeStr=boolean  SampleTime=7.65403750478377e-09
  concatenate : Concatenate  NumInputs=10
  crp_out_delay : Delay  DelayLength=double(1)  InitialCondition=0  SampleTime=7.65403750478377e-09
  dtc : hdlmdlgenlib/Buffer
  dtc1 : hdlmdlgenlib/Buffer
  in0_repeat : RateTransition  Integrity=off  Deterministic=off  OutPortSampleTimeOpt=Multiple of input port sample time  OutPortSampleTimeMultiple=1/67
  in1_repeat : RateTransition  Integrity=off  Deterministic=off  OutPortSampleTimeOpt=Multiple of input port sample time  OutPortSampleTimeMultiple=1/67
  rd_{0..1,3..5} (5 alike) : Delay  DelayLength=double(1)  InitialCondition=0  SampleTime=7.65403750478377e-09
  rd_2 : Delay  DelayLength=double(2)  InitialCondition=0  SampleTime=7.65403750478377e-09
  sumOuputEqnComp : Sum  OutDataTypeStr=fixdt(1, 25, 13)  SampleTime=7.65403750478377e-09
  sumStateEqnComp : Sum  OutDataTypeStr=fixdt(1, 25, 13)  SampleTime=7.65403750478377e-09
  t : Demux  Outputs=20
  I_load : Outport  SampleTime=7.65403750478377e-09
  is_out_MOSFET : Outport  Port=2  SampleTime=7.65403750478377e-09
  vs_out_MOSFET : Outport  Port=3  SampleTime=7.65403750478377e-09
  is_out_MOSFET1 : Outport  Port=4  SampleTime=7.65403750478377e-09
  vs_out_MOSFET1 : Outport  Port=5  SampleTime=7.65403750478377e-09
  is_out_MOSFET2 : Outport  Port=6  SampleTime=7.65403750478377e-09
  vs_out_MOSFET2 : Outport  Port=7  SampleTime=7.65403750478377e-09
  is_out_MOSFET3 : Outport  Port=8  SampleTime=7.65403750478377e-09
  vs_out_MOSFET3 : Outport  Port=9  SampleTime=7.65403750478377e-09
  is_out_MOSFET4 : Outport  Port=10  SampleTime=7.65403750478377e-09
  vs_out_MOSFET4 : Outport  Port=11  SampleTime=7.65403750478377e-09
  is_out_MOSFET5 : Outport  Port=12  SampleTime=7.65403750478377e-09
  vs_out_MOSFET5 : Outport  Port=13  SampleTime=7.65403750478377e-09
  Vout : Outport  Port=14  SampleTime=7.65403750478377e-09
  Ib : Outport  Port=15  SampleTime=7.65403750478377e-09
  Ic : Outport  Port=16  SampleTime=7.65403750478377e-09
  Ia : Outport  Port=17  SampleTime=7.65403750478377e-09
  Vb : Outport  Port=18  SampleTime=7.65403750478377e-09
  Vc : Outport  Port=19  SampleTime=7.65403750478377e-09
  Va : Outport  Port=20  SampleTime=7.65403750478377e-09
  wires:
  ic_in_MOSFET3/1 -> concatenate/5
  I_load_in/1 -> concatenate/1
  crp_out_delay/1 -> State/1
  ic_in_MOSFET4/1 -> concatenate/6
  t/1 -> I_load/1
  ic_in_MOSFET/1 -> concatenate/2
  ic_in_MOSFET1/1 -> concatenate/3
  Data Type Conversion/1 -> Sparse Matrix-Vector Product3/1(in0), Sparse Matrix-Vector Product/1(in0)
  ic_in_MOSFET2/1 -> concatenate/4
  t/16 -> Ic/1
  Sparse Matrix-Vector Product2/1(matrixCOutSignal) -> rd_3/1
  ic_in_MOSFET5/1 -> concatenate/7
  va/1 -> concatenate/8
  State/1 -> State_absorbed/1
  vb/1 -> concatenate/9
  t/13 -> vs_out_MOSFET5/1
  t/9 -> vs_out_MOSFET3/1
  vc/1 -> concatenate/10
  concatenate/1 -> Data Type Conversion/1
  t/10 -> is_out_MOSFET4/1
  Zero3/1 -> Sparse Matrix-Vector Product3/2(selectSignal)
  rd_1/1 -> State_switch/2
  Zero/1 -> Sparse Matrix-Vector Product/2(selectSignal)
  t/20 -> Va/1
  t/15 -> Ib/1
  sch_ctr_66/1 -> Sparse Matrix-Vector Product2/3(enb_counter), Sparse Matrix-Vector Product1/3(enb_counter), Sparse Matrix-Vector Product3/3(enb_counter), Sparse Matrix-Vector Product/3(enb_counter)
  Sparse Matrix-Vector Product3/1(matrixDOutSignal) -> rd_2/1
  Sparse Matrix-Vector Product/1(matrixBOutSignal) -> rd_4/1
  in1_repeat/1 -> rd_1/1
  rd_4/1 -> sumStateEqnComp/1
  rd_2/1 -> sumOuputEqnComp/1
  rd_0/1 -> State_switch/1
  sumStateEqnComp/1 -> dtc1/1
  t/11 -> vs_out_MOSFET4/1
  sumOuputEqnComp/1 -> dtc/1
  dtc1/1 -> crp_out_delay/1
  State_ctrl_const/1 -> State_ctrl_delay/1
  State_absorbed/1 -> in0_repeat/1
  Zero1/1 -> Sparse Matrix-Vector Product1/2(selectSignal)
  State_ctrl_delay/1 -> in1_repeat/1
  in0_repeat/1 -> rd_0/1
  t/7 -> vs_out_MOSFET2/1
  State_Initial_Val/1 -> State_switch/3
  Sparse Matrix-Vector Product1/1(matrixAOutSignal) -> rd_5/1
  State_switch/1 -> Sparse Matrix-Vector Product1/1(delayOutSignal), Sparse Matrix-Vector Product2/1(delayOutSignal)
  Zero2/1 -> Sparse Matrix-Vector Product2/2(selectSignal)
  Data Type Conversion1/1 -> t/1
  rd_5/1 -> sumStateEqnComp/2
  t/6 -> is_out_MOSFET2/1
  rd_3/1 -> sumOuputEqnComp/2
  dtc/1 -> Data Type Conversion1/1
  t/2 -> is_out_MOSFET/1
  t/3 -> vs_out_MOSFET/1
  t/4 -> is_out_MOSFET1/1
  t/5 -> vs_out_MOSFET1/1
  t/8 -> is_out_MOSFET3/1
  t/12 -> is_out_MOSFET5/1
  t/14 -> Vout/1
  t/17 -> Ia/1
  t/18 -> Vb/1
  t/19 -> Vc/1

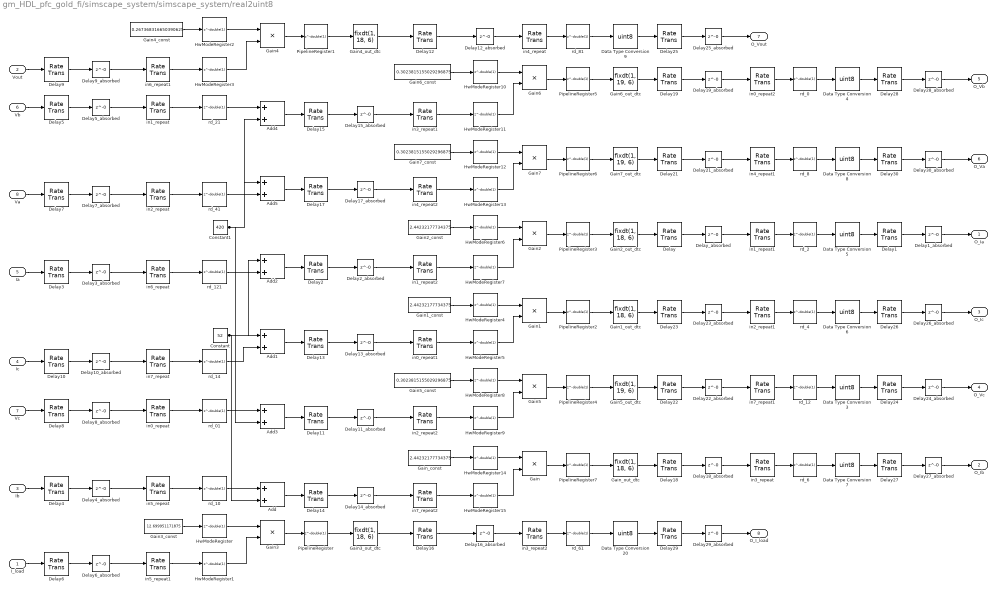
== system gm_HDL_pfc_gold_fi/simscape_system/simscape_system/real2uint8 ==
  I_load : Inport  OutDataTypeStr=fixdt(1, 18, 6)  PortDimensions=1  SampleTime=7.65403750478377e-09
  Vout : Inport  Port=2  OutDataTypeStr=fixdt(1, 18, 6)  PortDimensions=1  SampleTime=7.65403750478377e-09
  Ib : Inport  Port=3  OutDataTypeStr=fixdt(1, 18, 6)  PortDimensions=1  SampleTime=7.65403750478377e-09
  Ic : Inport  Port=4  OutDataTypeStr=fixdt(1, 18, 6)  PortDimensions=1  SampleTime=7.65403750478377e-09
  Ia : Inport  Port=5  OutDataTypeStr=fixdt(1, 18, 6)  PortDimensions=1  SampleTime=7.65403750478377e-09
  Vb : Inport  Port=6  OutDataTypeStr=fixdt(1, 18, 6)  PortDimensions=1  SampleTime=7.65403750478377e-09
  Vc : Inport  Port=7  OutDataTypeStr=fixdt(1, 18, 6)  PortDimensions=1  SampleTime=7.65403750478377e-09
  Va : Inport  Port=8  OutDataTypeStr=fixdt(1, 18, 6)  PortDimensions=1  SampleTime=7.65403750478377e-09
  Add : Sum  OutDataTypeStr=fixdt(1, 18, 6)  AccumDataTypeStr=fixdt(1, 19, 6)  SampleTime=7.65403750478377e-09
  Add1 : Sum  OutDataTypeStr=fixdt(1, 18, 6)  AccumDataTypeStr=fixdt(1, 19, 6)  SampleTime=7.65403750478377e-09
  Add2 : Sum  OutDataTypeStr=fixdt(1, 18, 6)  AccumDataTypeStr=fixdt(1, 19, 6)  SampleTime=7.65403750478377e-09
  Add3 : Sum  OutDataTypeStr=fixdt(1, 19, 6)  AccumDataTypeStr=fixdt(1, 19, 6)  SampleTime=7.65403750478377e-09
  Add4 : Sum  OutDataTypeStr=fixdt(1, 19, 6)  AccumDataTypeStr=fixdt(1, 19, 6)  SampleTime=7.65403750478377e-09
  Add5 : Sum  OutDataTypeStr=fixdt(1, 19, 6)  AccumDataTypeStr=fixdt(1, 19, 6)  SampleTime=7.65403750478377e-09
  Constant : Constant  Value=52  OutDataTypeStr=fixdt(1, 18, 6)  SampleTime=7.65403750478377e-09
  Constant1 : Constant  Value=420  OutDataTypeStr=fixdt(1, 18, 6)  SampleTime=7.65403750478377e-09
  Data Type Conversion{3..9,20} (8 alike) : DataTypeConversion  OutDataTypeStr=uint8  RndMeth=Nearest  SampleTime=7.65403750478377e-09  SaturateOnIntegerOverflow=off
  Delay{,1..19,21..30} (30 alike) : RateTransition  InitialCondition=double(0)  OutPortSampleTimeOpt=Multiple of input port sample time  OutPortSampleTimeMultiple=67
  Delay10_absorbed : Delay  DelayLength=0
  Delay11_absorbed : Delay  DelayLength=0
  Delay12_absorbed : Delay  DelayLength=0
  Delay13_absorbed : Delay  DelayLength=0
  Delay14_absorbed : Delay  DelayLength=0
  Delay15_absorbed : Delay  DelayLength=0
  Delay16_absorbed : Delay  DelayLength=0
  Delay17_absorbed : Delay  DelayLength=0
  Delay18_absorbed : Delay  DelayLength=0
  Delay19_absorbed : Delay  DelayLength=0
  Delay1_absorbed : Delay  DelayLength=0
  Delay21_absorbed : Delay  DelayLength=0
  Delay22_absorbed : Delay  DelayLength=0
  Delay23_absorbed : Delay  DelayLength=0
  Delay24_absorbed : Delay  DelayLength=0
  Delay25_absorbed : Delay  DelayLength=0
  Delay26_absorbed : Delay  DelayLength=0
  Delay27_absorbed : Delay  DelayLength=0
  Delay28_absorbed : Delay  DelayLength=0
  Delay29_absorbed : Delay  DelayLength=0
  Delay2_absorbed : Delay  DelayLength=0
  Delay30_absorbed : Delay  DelayLength=0
  Delay3_absorbed : Delay  DelayLength=0
  Delay4_absorbed : Delay  DelayLength=0
  Delay5_absorbed : Delay  DelayLength=0
  Delay6_absorbed : Delay  DelayLength=0
  Delay7_absorbed : Delay  DelayLength=0
  Delay8_absorbed : Delay  DelayLength=0
  Delay9_absorbed : Delay  DelayLength=0
  Delay_absorbed : Delay  DelayLength=0
  Gain : Product  Inputs=**  OutDataTypeStr=fixdt(1, 36, 21)  SampleTime=7.65403750478377e-09
  Gain1 : Product  Inputs=**  OutDataTypeStr=fixdt(1, 36, 21)  SampleTime=7.65403750478377e-09
  Gain1_const : Constant  Value=2.44232177734375  OutDataTypeStr=fixdt(1, 18, 15)  SampleTime=7.65403750478377e-09
  Gain1_out_dtc : DataTypeConversion  OutDataTypeStr=fixdt(1, 18, 6)  SampleTime=7.65403750478377e-09  SaturateOnIntegerOverflow=off  RndMeth=Floor
  Gain2 : Product  Inputs=**  OutDataTypeStr=fixdt(1, 36, 21)  SampleTime=7.65403750478377e-09
  Gain2_const : Constant  Value=2.44232177734375  OutDataTypeStr=fixdt(1, 18, 15)  SampleTime=7.65403750478377e-09
  Gain2_out_dtc : DataTypeConversion  OutDataTypeStr=fixdt(1, 18, 6)  SampleTime=7.65403750478377e-09  SaturateOnIntegerOverflow=off  RndMeth=Floor
  Gain3 : Product  Inputs=**  OutDataTypeStr=fixdt(1, 36, 19)  SampleTime=7.65403750478377e-09
  Gain3_const : Constant  Value=12.699951171875  OutDataTypeStr=fixdt(1, 18, 13)  SampleTime=7.65403750478377e-09
  Gain3_out_dtc : DataTypeConversion  OutDataTypeStr=fixdt(1, 18, 6)  SampleTime=7.65403750478377e-09  SaturateOnIntegerOverflow=off  RndMeth=Floor
  Gain4 : Product  Inputs=**  OutDataTypeStr=fixdt(1, 36, 24)  SampleTime=7.65403750478377e-09
  Gain4_const : Constant  Value=0.267368316650390625  OutDataTypeStr=fixdt(1, 18, 18)  SampleTime=7.65403750478377e-09
  Gain4_out_dtc : DataTypeConversion  OutDataTypeStr=fixdt(1, 18, 6)  SampleTime=7.65403750478377e-09  SaturateOnIntegerOverflow=off  RndMeth=Floor
  Gain5 : Product  Inputs=**  OutDataTypeStr=fixdt(1, 38, 25)  SampleTime=7.65403750478377e-09
  Gain5_const : Constant  Value=0.3023815155029296875  OutDataTypeStr=fixdt(1, 19, 19)  SampleTime=7.65403750478377e-09
  Gain5_out_dtc : DataTypeConversion  OutDataTypeStr=fixdt(1, 19, 6)  SampleTime=7.65403750478377e-09  SaturateOnIntegerOverflow=off  RndMeth=Floor
  Gain6 : Product  Inputs=**  OutDataTypeStr=fixdt(1, 38, 25)  SampleTime=7.65403750478377e-09
  Gain6_const : Constant  Value=0.3023815155029296875  OutDataTypeStr=fixdt(1, 19, 19)  SampleTime=7.65403750478377e-09
  Gain6_out_dtc : DataTypeConversion  OutDataTypeStr=fixdt(1, 19, 6)  SampleTime=7.65403750478377e-09  SaturateOnIntegerOverflow=off  RndMeth=Floor
  Gain7 : Product  Inputs=**  OutDataTypeStr=fixdt(1, 38, 25)  SampleTime=7.65403750478377e-09
  Gain7_const : Constant  Value=0.3023815155029296875  OutDataTypeStr=fixdt(1, 19, 19)  SampleTime=7.65403750478377e-09
  Gain7_out_dtc : DataTypeConversion  OutDataTypeStr=fixdt(1, 19, 6)  SampleTime=7.65403750478377e-09  SaturateOnIntegerOverflow=off  RndMeth=Floor
  Gain_const : Constant  Value=2.44232177734375  OutDataTypeStr=fixdt(1, 18, 15)  SampleTime=7.65403750478377e-09
  Gain_out_dtc : DataTypeConversion  OutDataTypeStr=fixdt(1, 18, 6)  SampleTime=7.65403750478377e-09  SaturateOnIntegerOverflow=off  RndMeth=Floor
  HwModeRegister{,1..15} (16 alike) : Delay  DelayLength=double(1)  InitialCondition=0  SampleTime=7.65403750478377e-09
  PipelineRegister{,1..7} (8 alike) : Delay  DelayLength=double(1)  InitialCondition=0  SampleTime=7.65403750478377e-09
  in0_repeat : RateTransition  Integrity=off  Deterministic=off  OutPortSampleTimeOpt=Multiple of input port sample time  OutPortSampleTimeMultiple=1/67
  in0_repeat1 : RateTransition  Integrity=off  Deterministic=off  OutPortSampleTimeOpt=Multiple of input port sample time  OutPortSampleTimeMultiple=1/67
  in0_repeat2 : RateTransition  Integrity=off  Deterministic=off  OutPortSampleTimeOpt=Multiple of input port sample time  OutPortSampleTimeMultiple=1/67
  in1_repeat : RateTransition  Integrity=off  Deterministic=off  OutPortSampleTimeOpt=Multiple of input port sample time  OutPortSampleTimeMultiple=1/67
  in1_repeat1 : RateTransition  Integrity=off  Deterministic=off  OutPortSampleTimeOpt=Multiple of input port sample time  OutPortSampleTimeMultiple=1/67
  in1_repeat2 : RateTransition  Integrity=off  Deterministic=off  OutPortSampleTimeOpt=Multiple of input port sample time  OutPortSampleTimeMultiple=1/67
  in2_repeat : RateTransition  Integrity=off  Deterministic=off  OutPortSampleTimeOpt=Multiple of input port sample time  OutPortSampleTimeMultiple=1/67
  in2_repeat1 : RateTransition  Integrity=off  Deterministic=off  OutPortSampleTimeOpt=Multiple of input port sample time  OutPortSampleTimeMultiple=1/67
  in2_repeat2 : RateTransition  Integrity=off  Deterministic=off  OutPortSampleTimeOpt=Multiple of input port sample time  OutPortSampleTimeMultiple=1/67
  in3_repeat : RateTransition  Integrity=off  Deterministic=off  OutPortSampleTimeOpt=Multiple of input port sample time  OutPortSampleTimeMultiple=1/67
  in3_repeat1 : RateTransition  Integrity=off  Deterministic=off  OutPortSampleTimeOpt=Multiple of input port sample time  OutPortSampleTimeMultiple=1/67
  in3_repeat2 : RateTransition  Integrity=off  Deterministic=off  OutPortSampleTimeOpt=Multiple of input port sample time  OutPortSampleTimeMultiple=1/67
  in4_repeat : RateTransition  Integrity=off  Deterministic=off  OutPortSampleTimeOpt=Multiple of input port sample time  OutPortSampleTimeMultiple=1/67
  in4_repeat1 : RateTransition  Integrity=off  Deterministic=off  OutPortSampleTimeOpt=Multiple of input port sample time  OutPortSampleTimeMultiple=1/67
  in4_repeat2 : RateTransition  Integrity=off  Deterministic=off  OutPortSampleTimeOpt=Multiple of input port sample time  OutPortSampleTimeMultiple=1/67
  in5_repeat : RateTransition  Integrity=off  Deterministic=off  OutPortSampleTimeOpt=Multiple of input port sample time  OutPortSampleTimeMultiple=1/67
  in5_repeat1 : RateTransition  Integrity=off  Deterministic=off  OutPortSampleTimeOpt=Multiple of input port sample time  OutPortSampleTimeMultiple=1/67
  in6_repeat : RateTransition  Integrity=off  Deterministic=off  OutPortSampleTimeOpt=Multiple of input port sample time  OutPortSampleTimeMultiple=1/67
  in6_repeat1 : RateTransition  Integrity=off  Deterministic=off  OutPortSampleTimeOpt=Multiple of input port sample time  OutPortSampleTimeMultiple=1/67
  in7_repeat : RateTransition  Integrity=off  Deterministic=off  OutPortSampleTimeOpt=Multiple of input port sample time  OutPortSampleTimeMultiple=1/67
  in7_repeat1 : RateTransition  Integrity=off  Deterministic=off  OutPortSampleTimeOpt=Multiple of input port sample time  OutPortSampleTimeMultiple=1/67
  in7_repeat2 : RateTransition  Integrity=off  Deterministic=off  OutPortSampleTimeOpt=Multiple of input port sample time  OutPortSampleTimeMultiple=1/67
  rd_{0,2,4,6,8,10,12,14,21,41,61,81,121} (13 alike) : Delay  DelayLength=double(1)  InitialCondition=0  SampleTime=7.65403750478377e-09
  rd_01 : Delay  DelayLength=double(1)  InitialCondition=0  SampleTime=7.65403750478377e-09
  O_Ia : Outport  SampleTime=5.12820512820513e-07
  O_Ib : Outport  Port=2  SampleTime=5.12820512820513e-07
  O_Ic : Outport  Port=3  SampleTime=5.12820512820513e-07
  O_Vc : Outport  Port=4  SampleTime=5.12820512820513e-07
  O_Vb : Outport  Port=5  SampleTime=5.12820512820513e-07
  O_Va : Outport  Port=6  SampleTime=5.12820512820513e-07
  O_Vout : Outport  Port=7  SampleTime=5.12820512820513e-07
  O_I_load : Outport  Port=8  SampleTime=5.12820512820513e-07
  wires:
  Gain4_const/1 -> HwModeRegister2/1
  Gain2_const/1 -> HwModeRegister6/1
  HwModeRegister10/1 -> Gain6/1
  HwModeRegister15/1 -> Gain/2
  rd_12/1 -> Data Type Conversion3/1
  rd_21/1 -> Add4/1
  Delay2/1 -> Delay2_absorbed/1
  HwModeRegister11/1 -> Gain6/2
  HwModeRegister6/1 -> Gain2/1
  Constant/1 -> Add/2, Add1/1, Add2/1
  HwModeRegister14/1 -> Gain/1
  Gain/1 -> PipelineRegister7/1
  Gain1/1 -> PipelineRegister2/1
  PipelineRegister3/1 -> Gain2_out_dtc/1
  Delay8/1 -> Delay8_absorbed/1
  Gain7/1 -> PipelineRegister6/1
  HwModeRegister9/1 -> Gain5/2
  Delay10_absorbed/1 -> in7_repeat/1
  HwModeRegister13/1 -> Gain7/2
  Delay_absorbed/1 -> in1_repeat1/1
  in1_repeat2/1 -> HwModeRegister7/1
  HwModeRegister12/1 -> Gain7/1
  HwModeRegister5/1 -> Gain1/2
  HwModeRegister8/1 -> Gain5/1
  PipelineRegister6/1 -> Gain7_out_dtc/1
  HwModeRegister2/1 -> Gain4/1
  rd_8/1 -> Data Type Conversion8/1
  Delay9/1 -> Delay9_absorbed/1
  Gain6/1 -> PipelineRegister5/1
  Vc/1 -> Delay8/1
  Gain6_const/1 -> HwModeRegister10/1
  PipelineRegister/1 -> Gain3_out_dtc/1
  rd_0/1 -> Data Type Conversion4/1
  Gain1_const/1 -> HwModeRegister4/1
  Delay3_absorbed/1 -> in6_repeat/1
  Delay19_absorbed/1 -> in0_repeat2/1
  Delay17/1 -> Delay17_absorbed/1
  rd_14/1 -> Add1/2
  Gain5/1 -> PipelineRegister4/1
  in0_repeat2/1 -> rd_0/1
  HwModeRegister7/1 -> Gain2/2
  rd_2/1 -> Data Type Conversion5/1
  PipelineRegister1/1 -> Gain4_out_dtc/1
  rd_4/1 -> Data Type Conversion6/1
  Gain2/1 -> PipelineRegister3/1
  in7_repeat1/1 -> rd_12/1
  HwModeRegister4/1 -> Gain1/1
  rd_121/1 -> Add2/2
  rd_01/1 -> Add3/1
  Gain_const/1 -> HwModeRegister14/1
  HwModeRegister3/1 -> Gain4/2
  Gain4/1 -> PipelineRegister1/1
  Gain3_out_dtc/1 -> Delay16/1
  Gain5_const/1 -> HwModeRegister8/1
  Vout/1 -> Delay9/1
  Delay22/1 -> Delay22_absorbed/1
  HwModeRegister1/1 -> Gain3/2
  PipelineRegister5/1 -> Gain6_out_dtc/1
  Delay25/1 -> Delay25_absorbed/1
  rd_61/1 -> Data Type Conversion20/1
  Delay16/1 -> Delay16_absorbed/1
  Delay14_absorbed/1 -> in7_repeat2/1
  Gain7_const/1 -> HwModeRegister12/1
  HwModeRegister/1 -> Gain3/1
  Gain3/1 -> PipelineRegister/1
  Delay19/1 -> Delay19_absorbed/1
  Delay13/1 -> Delay13_absorbed/1
  Data Type Conversion8/1 -> Delay30/1
  rd_10/1 -> Add/1
  rd_41/1 -> Add5/2
  Delay26/1 -> Delay26_absorbed/1
  PipelineRegister7/1 -> Gain_out_dtc/1
  Gain7_out_dtc/1 -> Delay21/1
  rd_81/1 -> Data Type Conversion9/1
  PipelineRegister4/1 -> Gain5_out_dtc/1
  Gain_out_dtc/1 -> Delay18/1
  PipelineRegister2/1 -> Gain1_out_dtc/1
  Delay3/1 -> Delay3_absorbed/1
  rd_6/1 -> Data Type Conversion7/1
  in2_repeat/1 -> rd_41/1
  Gain3_const/1 -> HwModeRegister/1
  Delay16_absorbed/1 -> in3_repeat2/1
  in0_repeat1/1 -> HwModeRegister5/1
  Delay13_absorbed/1 -> in0_repeat1/1
  Delay2_absorbed/1 -> in1_repeat2/1
  in2_repeat2/1 -> HwModeRegister9/1
  in5_repeat/1 -> rd_10/1
  Delay/1 -> Delay_absorbed/1
  Delay11_absorbed/1 -> in2_repeat2/1
  Delay27/1 -> Delay27_absorbed/1
  Delay11/1 -> Delay11_absorbed/1
  in3_repeat1/1 -> HwModeRegister11/1
  Delay15_absorbed/1 -> in3_repeat1/1
  Delay15/1 -> Delay15_absorbed/1
  in4_repeat2/1 -> HwModeRegister13/1
  Delay17_absorbed/1 -> in4_repeat2/1
  Delay6_absorbed/1 -> in5_repeat1/1
  in7_repeat2/1 -> HwModeRegister15/1
  Delay14/1 -> Delay14_absorbed/1
  Add/1 -> Delay14/1
  Constant1/1 -> Add5/1, Add4/2, Add3/2
  in1_repeat1/1 -> rd_2/1
  in2_repeat1/1 -> rd_4/1
  Delay23_absorbed/1 -> in2_repeat1/1
  Ic/1 -> Delay10/1
  Delay23/1 -> Delay23_absorbed/1
  in3_repeat/1 -> rd_6/1
  Delay18_absorbed/1 -> in3_repeat/1
  Delay18/1 -> Delay18_absorbed/1
  Delay10/1 -> Delay10_absorbed/1
  in4_repeat1/1 -> rd_8/1
  Delay21_absorbed/1 -> in4_repeat1/1
  Delay30_absorbed/1 -> O_Va/1
  Delay21/1 -> Delay21_absorbed/1
  in5_repeat1/1 -> HwModeRegister1/1
  Delay6/1 -> Delay6_absorbed/1
  in6_repeat1/1 -> HwModeRegister3/1
  in0_repeat/1 -> rd_01/1
  Delay9_absorbed/1 -> in6_repeat1/1
  Gain6_out_dtc/1 -> Delay19/1
  Gain5_out_dtc/1 -> Delay22/1
  Gain2_out_dtc/1 -> Delay/1
  Gain1_out_dtc/1 -> Delay23/1
  Delay22_absorbed/1 -> in7_repeat1/1
  Gain4_out_dtc/1 -> Delay12/1
  Delay12_absorbed/1 -> in4_repeat/1
  Add4/1 -> Delay15/1
  Delay12/1 -> Delay12_absorbed/1
  in3_repeat2/1 -> rd_61/1
  in4_repeat/1 -> rd_81/1
  I_load/1 -> Delay6/1
  in7_repeat/1 -> rd_14/1
  in6_repeat/1 -> rd_121/1
  in1_repeat/1 -> rd_21/1
  Add1/1 -> Delay13/1
  Add2/1 -> Delay2/1
  Add5/1 -> Delay17/1
  Add3/1 -> Delay11/1
  Va/1 -> Delay7/1
  Delay28_absorbed/1 -> O_Vb/1
  Delay8_absorbed/1 -> in0_repeat/1
  Delay7_absorbed/1 -> in2_repeat/1
  Delay5_absorbed/1 -> in1_repeat/1
  Delay4_absorbed/1 -> in5_repeat/1
  Delay7/1 -> Delay7_absorbed/1
  Delay5/1 -> Delay5_absorbed/1
  Delay4/1 -> Delay4_absorbed/1
  Delay29/1 -> Delay29_absorbed/1
  Data Type Conversion20/1 -> Delay29/1
  Delay24_absorbed/1 -> O_Vc/1
  Delay27_absorbed/1 -> O_Ib/1
  Delay26_absorbed/1 -> O_Ic/1
  Delay1_absorbed/1 -> O_Ia/1
  Delay24/1 -> Delay24_absorbed/1
  Delay30/1 -> Delay30_absorbed/1
  Delay28/1 -> Delay28_absorbed/1
  Delay1/1 -> Delay1_absorbed/1
  Data Type Conversion3/1 -> Delay24/1
  Data Type Conversion7/1 -> Delay27/1
  Data Type Conversion6/1 -> Delay26/1
  Data Type Conversion5/1 -> Delay1/1
  Data Type Conversion4/1 -> Delay28/1
  Delay25_absorbed/1 -> O_Vout/1
  Delay29_absorbed/1 -> O_I_load/1
  Data Type Conversion9/1 -> Delay25/1
  Vb/1 -> Delay5/1
  Ia/1 -> Delay3/1
  Ib/1 -> Delay4/1
